simulink model "Airship_Model_2"  (R2020a)
settings: Solver=VariableStepAuto  StartTime=0.0  StopTime=300  RelTol=1e-3
values from neighbouring files (symbols this model uses):
  d = [0; 0; 0; 0; 0; 0; 0; 0; 0; 0; 0; 0]    [Inputs.m]
  g = 9.81    [Inputs.m]
  M = 997    [Inputs.m]
  rho = 0.8891    [Inputs.m]
  Sref = 6515.77    [Inputs.m]
  x0 = [0; 0; 0; 0; 0; 0; 0; 0; -20; 0; 0; 0]    [Inputs.m]
undefined symbols (not defined in the file or in its folder): sigbuilder_block
libraries: simulink x4
settings Model: Creator=roohan  LastModifiedBy=HP

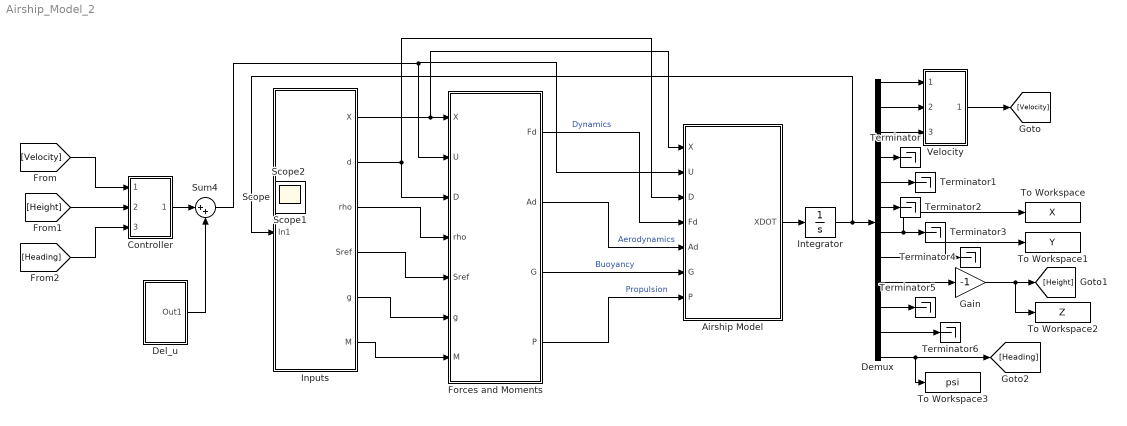
== system Airship_Model_2 ==
  Airship Model : MATLAB Function  TreatAsAtomicUnit=on
  Controller : Subsystem
  Del_u : Subsystem
  Demux : Demux  Outputs=12
  Forces and Moments : Subsystem
  Gain : Gain  Gain=-1
  Inputs : Subsystem
  Integrator : Integrator
  Sum4 : Sum  Inputs=|++
  Terminator{,1..6} (7 alike) : Terminator
  To Workspace : ToWorkspace  VariableName=X  SaveFormat=Timeseries  SampleTime=-1
  To Workspace1 : ToWorkspace  VariableName=Y  SaveFormat=Timeseries  SampleTime=-1
  To Workspace2 : ToWorkspace  VariableName=Z  SaveFormat=Timeseries  SampleTime=-1
  To Workspace3 : ToWorkspace  VariableName=psi  SaveFormat=Timeseries  SampleTime=-1
  Velocity : Subsystem
  Scope : Scope
  Scope1 : Scope
  Scope2 : Scope
  wires:
  Airship Model/1(XDOT) -> Integrator/1
  Integrator/1 -> Inputs/1(In1), Demux/1
  Forces and Moments/1(Fd) -> Airship Model/4(Fd)  "Dynamics"
  Forces and Moments/2(Ad) -> Airship Model/5(Ad)  "Aerodynamics"
  Forces and Moments/3(G) -> Airship Model/6(G)  "Buoyancy"
  Forces and Moments/4(P) -> Airship Model/7(P)  "Propulsion"
  Inputs/2(d) -> Forces and Moments/3(D), Airship Model/3(D)
  Inputs/3(rho) -> Forces and Moments/4(rho)
  Inputs/4(Sref) -> Forces and Moments/5(Sref)
  Inputs/5(g) -> Forces and Moments/6(g)
  Inputs/6(M) -> Forces and Moments/7(M)
  Inputs/1(X) -> Forces and Moments/1(X), Airship Model/1(X)
  Demux/9 -> Gain/1
  Gain/1 -> [Height], To Workspace2/1
  Demux/12 -> To Workspace3/1, [Heading]
  Sum4/1 -> Airship Model/2(U), Forces and Moments/2(U)
  Del_u/1(Out1) -> Sum4/2
  [Velocity] -> Controller/1(In1)
  [Height] -> Controller/2(In2)
  [Heading] -> Controller/3(In3)
  Controller/1(Out1) -> Sum4/1
  Demux/4 -> Terminator/1
  Demux/5 -> Terminator1/1
  Demux/6 -> Terminator2/1
  Demux/7 -> To Workspace/1, Terminator3/1
  Demux/8 -> To Workspace1/1, Terminator4/1
  Demux/10 -> Terminator5/1
  Demux/11 -> Terminator6/1
  Demux/1 -> Velocity/1(In1)
  Demux/2 -> Velocity/2(In2)
  Demux/3 -> Velocity/3(In3)
  Velocity/1(Out1) -> [Velocity]

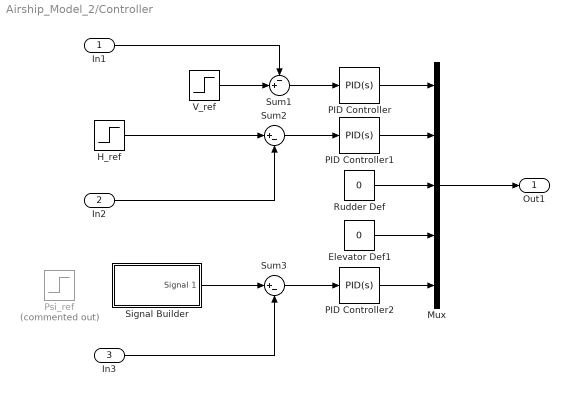
== system Airship_Model_2/Controller ==
  In1 : Inport
  In2 : Inport  Port=2
  In3 : Inport  Port=3
  Elevator Def1 : Constant  Value=0
  H_ref : Step  SampleTime=0.075
  Mux : Mux  Inputs=5
  PID Controller : simulink/Continuous/PID Controller  Controller=PID  Form=Parallel  TimeDomain=Continuous-time  UseExternalTs=off  SampleTime=-1  IntegratorMethod=Forward Euler  FilterMethod=Forward Euler  ControllerParametersSource=internal  P=15  I=0.001  D=15  UseFilter=on  N=100  TunerSelectOption=Transfer Function Based (PID Tuner App)  InitialConditionSource=internal  InitialConditionForIntegrator=0  InitialConditionForFilter=0  DifferentiatorICPrevScaledInput=0  ExternalReset=none  TrackingMode=off  Kt=1  LimitOutput=off  UpperSaturationLimit=inf  LowerSaturationLimit=-inf  LinearizeAsGain=on  AntiWindupMode=none  Kb=1  POutMin=[]  POutMax=[]  IOutMin=[]  IOutMax=[]  DOutMin=[]  DOutMax=[]  NOutMin=[]  NOutMax=[]  SumOutMin=[]  SumOutMax=[]  SaturationOutMin=[]  SaturationOutMax=[]  PParamMin=[]  PParamMax=[]  IParamMin=[]  IParamMax=[]  DParamMin=[]  DParamMax=[]  NParamMin=[]  NParamMax=[]  KbParamMin=[]  KbParamMax=[]  KtParamMin=[]  KtParamMax=[]  KbOutMin=[]  KbOutMax=[]  KtOutMin=[]  KtOutMax=[]  IntegratorOutMin=[]  IntegratorOutMax=[]  FilterOutMin=[]  FilterOutMax=[]  SumI1OutMin=[]  SumI1OutMax=[]  SumI2OutMin=[]  SumI2OutMax=[]  SumI3OutMin=[]  SumI3OutMax=[]  SumI4OutMin=[]  SumI4OutMax=[]  SumDOutMin=[]  SumDOutMax=[]  DifferentiatorOutMin=[]  DifferentiatorOutMax=[]  FilterDiffOutCoefMin=[]  FilterDiffOutCoefMax=[]  ReciprocalOutMin=[]  ReciprocalOutMax=[]  SumDenOutMin=[]  SumDenOutMax=[]  SumNumOutMin=[]  SumNumOutMax=[]  DivideOutMin=[]  DivideOutMax=[]  UdiffTsProdOutMin=[]  UdiffTsProdOutMax=[]  NTsProdOutMin=[]  NTsProdOutMax=[]  UintegralTsProdOutMin=[]  UintegralTsProdOutMax=[]  UngainTsProdOutMin=[]  UngainTsProdOutMax=[]  IntegratorContinuousStateAttributes=''  IntegratorStateMustResolveToSignalObject=off  IntegratorRTWStateStorageClass=Auto  FilterContinuousStateAttributes=''  FilterStateMustResolveToSignalObject=off  FilterRTWStateStorageClass=Auto  ParallelPVariant=InternalParameters  IdealPVariant=Disabled  IVariant=InternalParameters  DVariant=InternalParameters  IntegratorVariant=Continuous  SatVariant=Disabled  AWVariant=Passthrough  PCopyVariant=Disabled  TRVariant=Disabled  FdbkBlocksVariant=Forward  IdealPFdbkVariant=Disabled  SatFdbkVariant=Disabled  DerivativeFilterVariant=ContFilter  NVariant=InternalParameters  NCopyVariant=Disabled  FilterICVariant=InternalICsFilter  IntegratorICVariant=InternalICs  ExternalResetVariant=Disabled  TRSumVariant=Passthrough  SumFdbkVariant=Disabled  SumVariant=Sum_PID  TsampFilterVariant=InternalTs  TsampNgainVariant=Passthrough  TsampIntegralVariant=Passthrough
  PID Controller1 : simulink/Continuous/PID Controller  Controller=PID  Form=Parallel  TimeDomain=Continuous-time  UseExternalTs=off  SampleTime=-1  IntegratorMethod=Forward Euler  FilterMethod=Forward Euler  ControllerParametersSource=internal  P=3  I=0.005  D=10  UseFilter=on  N=100  TunerSelectOption=Transfer Function Based (PID Tuner App)  InitialConditionSource=internal  InitialConditionForIntegrator=0  InitialConditionForFilter=0  DifferentiatorICPrevScaledInput=0  ExternalReset=none  TrackingMode=off  Kt=1  LimitOutput=off  UpperSaturationLimit=inf  LowerSaturationLimit=-inf  LinearizeAsGain=on  AntiWindupMode=none  Kb=1  POutMin=[]  POutMax=[]  IOutMin=[]  IOutMax=[]  DOutMin=[]  DOutMax=[]  NOutMin=[]  NOutMax=[]  SumOutMin=[]  SumOutMax=[]  SaturationOutMin=[]  SaturationOutMax=[]  PParamMin=[]  PParamMax=[]  IParamMin=[]  IParamMax=[]  DParamMin=[]  DParamMax=[]  NParamMin=[]  NParamMax=[]  KbParamMin=[]  KbParamMax=[]  KtParamMin=[]  KtParamMax=[]  KbOutMin=[]  KbOutMax=[]  KtOutMin=[]  KtOutMax=[]  IntegratorOutMin=[]  IntegratorOutMax=[]  FilterOutMin=[]  FilterOutMax=[]  SumI1OutMin=[]  SumI1OutMax=[]  SumI2OutMin=[]  SumI2OutMax=[]  SumI3OutMin=[]  SumI3OutMax=[]  SumI4OutMin=[]  SumI4OutMax=[]  SumDOutMin=[]  SumDOutMax=[]  DifferentiatorOutMin=[]  DifferentiatorOutMax=[]  FilterDiffOutCoefMin=[]  FilterDiffOutCoefMax=[]  ReciprocalOutMin=[]  ReciprocalOutMax=[]  SumDenOutMin=[]  SumDenOutMax=[]  SumNumOutMin=[]  SumNumOutMax=[]  DivideOutMin=[]  DivideOutMax=[]  UdiffTsProdOutMin=[]  UdiffTsProdOutMax=[]  NTsProdOutMin=[]  NTsProdOutMax=[]  UintegralTsProdOutMin=[]  UintegralTsProdOutMax=[]  UngainTsProdOutMin=[]  UngainTsProdOutMax=[]  IntegratorContinuousStateAttributes=''  IntegratorStateMustResolveToSignalObject=off  IntegratorRTWStateStorageClass=Auto  FilterContinuousStateAttributes=''  FilterStateMustResolveToSignalObject=off  FilterRTWStateStorageClass=Auto  ParallelPVariant=InternalParameters  IdealPVariant=Disabled  IVariant=InternalParameters  DVariant=InternalParameters  IntegratorVariant=Continuous  SatVariant=Disabled  AWVariant=Passthrough  PCopyVariant=Disabled  TRVariant=Disabled  FdbkBlocksVariant=Forward  IdealPFdbkVariant=Disabled  SatFdbkVariant=Disabled  DerivativeFilterVariant=ContFilter  NVariant=InternalParameters  NCopyVariant=Disabled  FilterICVariant=InternalICsFilter  IntegratorICVariant=InternalICs  ExternalResetVariant=Disabled  TRSumVariant=Passthrough  SumFdbkVariant=Disabled  SumVariant=Sum_PID  TsampFilterVariant=InternalTs  TsampNgainVariant=Passthrough  TsampIntegralVariant=Passthrough
  PID Controller2 : simulink/Continuous/PID Controller  Controller=PID  Form=Parallel  TimeDomain=Continuous-time  UseExternalTs=off  SampleTime=-1  IntegratorMethod=Forward Euler  FilterMethod=Forward Euler  ControllerParametersSource=internal  P=-3  I=0  D=-7.5  UseFilter=on  N=100  TunerSelectOption=Transfer Function Based (PID Tuner App)  InitialConditionSource=internal  InitialConditionForIntegrator=0  InitialConditionForFilter=0  DifferentiatorICPrevScaledInput=0  ExternalReset=none  TrackingMode=off  Kt=1  LimitOutput=off  UpperSaturationLimit=inf  LowerSaturationLimit=-inf  LinearizeAsGain=on  AntiWindupMode=none  Kb=1  POutMin=[]  POutMax=[]  IOutMin=[]  IOutMax=[]  DOutMin=[]  DOutMax=[]  NOutMin=[]  NOutMax=[]  SumOutMin=[]  SumOutMax=[]  SaturationOutMin=[]  SaturationOutMax=[]  PParamMin=[]  PParamMax=[]  IParamMin=[]  IParamMax=[]  DParamMin=[]  DParamMax=[]  NParamMin=[]  NParamMax=[]  KbParamMin=[]  KbParamMax=[]  KtParamMin=[]  KtParamMax=[]  KbOutMin=[]  KbOutMax=[]  KtOutMin=[]  KtOutMax=[]  IntegratorOutMin=[]  IntegratorOutMax=[]  FilterOutMin=[]  FilterOutMax=[]  SumI1OutMin=[]  SumI1OutMax=[]  SumI2OutMin=[]  SumI2OutMax=[]  SumI3OutMin=[]  SumI3OutMax=[]  SumI4OutMin=[]  SumI4OutMax=[]  SumDOutMin=[]  SumDOutMax=[]  DifferentiatorOutMin=[]  DifferentiatorOutMax=[]  FilterDiffOutCoefMin=[]  FilterDiffOutCoefMax=[]  ReciprocalOutMin=[]  ReciprocalOutMax=[]  SumDenOutMin=[]  SumDenOutMax=[]  SumNumOutMin=[]  SumNumOutMax=[]  DivideOutMin=[]  DivideOutMax=[]  UdiffTsProdOutMin=[]  UdiffTsProdOutMax=[]  NTsProdOutMin=[]  NTsProdOutMax=[]  UintegralTsProdOutMin=[]  UintegralTsProdOutMax=[]  UngainTsProdOutMin=[]  UngainTsProdOutMax=[]  IntegratorContinuousStateAttributes=''  IntegratorStateMustResolveToSignalObject=off  IntegratorRTWStateStorageClass=Auto  FilterContinuousStateAttributes=''  FilterStateMustResolveToSignalObject=off  FilterRTWStateStorageClass=Auto  ParallelPVariant=InternalParameters  IdealPVariant=Disabled  IVariant=InternalParameters  DVariant=InternalParameters  IntegratorVariant=Continuous  SatVariant=Disabled  AWVariant=Passthrough  PCopyVariant=Disabled  TRVariant=Disabled  FdbkBlocksVariant=Forward  IdealPFdbkVariant=Disabled  SatFdbkVariant=Disabled  DerivativeFilterVariant=ContFilter  NVariant=InternalParameters  NCopyVariant=Disabled  FilterICVariant=InternalICsFilter  IntegratorICVariant=InternalICs  ExternalResetVariant=Disabled  TRSumVariant=Passthrough  SumFdbkVariant=Disabled  SumVariant=Sum_PID  TsampFilterVariant=InternalTs  TsampNgainVariant=Passthrough  TsampIntegralVariant=Passthrough
  Psi_ref : Step  Commented=on  After=1.57  SampleTime=1
  Rudder Def : Constant  Value=0
  Signal Builder : Subsystem  Tag=STV Subsys  LoadFcn=sigbuilder_block('load');  StartFcn=sigbuilder_block('start');  StopFcn=sigbuilder_block('stop');  ClipboardFcn=sigbuilder_block('clipboard');  mask(Sigbuilder block){tuvar=[0:10]}
      mask help: Simulink:masks:SigbuilderBlock_MD
      mask init:
      | if ~strcmp(get_param(bdroot(gcbh),'SimulationStatus'),'stopped') tuvar = sigbuilder_block('maskInit'); end
      settings: CopyFcn=sigbuilder_block('copy');  DeleteFcn=sigbuilder_block('delete');  ModelCloseFcn=sigbuilder_block('modelClose');  PreSaveFcn=sigbuilder_block('preSave');  PauseFcn=sigbuilder_block('pause');  ContinueFcn=sigbuilder_block('continue');  NameChangeFcn=sigbuilder_block('namechange');  OpenFcn=sigbuilder_block('open',[0 30 1024.5 488.25 ]);  CloseFcn=sigbuilder_block('close');
      mask Display: plot(0, 0, 100, 100,[2, 2, 32, 32, 2], [68, 8, 8, 68, 68],[32, 2], [38, 38], [32, 19, 2],[53, 60, 44], [32, 17, 17, 2],[16, 16, 31, 31]);txt = getActiveGroup(gcbh);text(2, 100, txt,'verticalAlignment', 'top');
  Sum1 : Sum  Inputs=-+|
  Sum2 : Sum  Inputs=|+-
  Sum3 : Sum  Inputs=|+-
  V_ref : Step  SampleTime=0.1
  Out1 : Outport
  wires:
  Sum2/1 -> PID Controller1/1
  Sum3/1 -> PID Controller2/1
  V_ref/1 -> Sum1/2
  PID Controller2/1 -> Mux/5
  PID Controller/1 -> Mux/1
  Rudder Def/1 -> Mux/3
  Sum1/1 -> PID Controller/1
  Elevator Def1/1 -> Mux/4
  PID Controller1/1 -> Mux/2
  In2/1 -> Sum2/2
  In1/1 -> Sum1/1
  In3/1 -> Sum3/2
  Mux/1 -> Out1/1
  Signal Builder/1(Signal 1) -> Sum3/1
  H_ref/1 -> Sum2/1

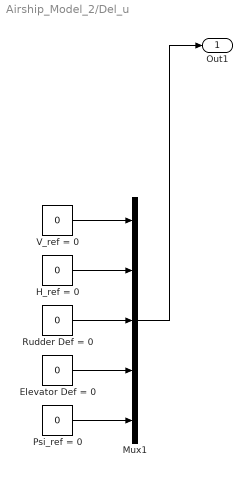
== system Airship_Model_2/Del_u ==
  Elevator Def = 0 : Constant  Value=0
  H_ref = 0 : Constant  Value=0
  Mux1 : Mux  Inputs=5
  Psi_ref = 0 : Constant  Value=0
  Rudder Def = 0 : Constant  Value=0
  V_ref = 0 : Constant  Value=0
  Out1 : Outport
  wires:
  V_ref = 0/1 -> Mux1/1
  H_ref = 0/1 -> Mux1/2
  Rudder Def = 0/1 -> Mux1/3
  Psi_ref = 0/1 -> Mux1/5
  Mux1/1 -> Out1/1
  Elevator Def = 0/1 -> Mux1/4

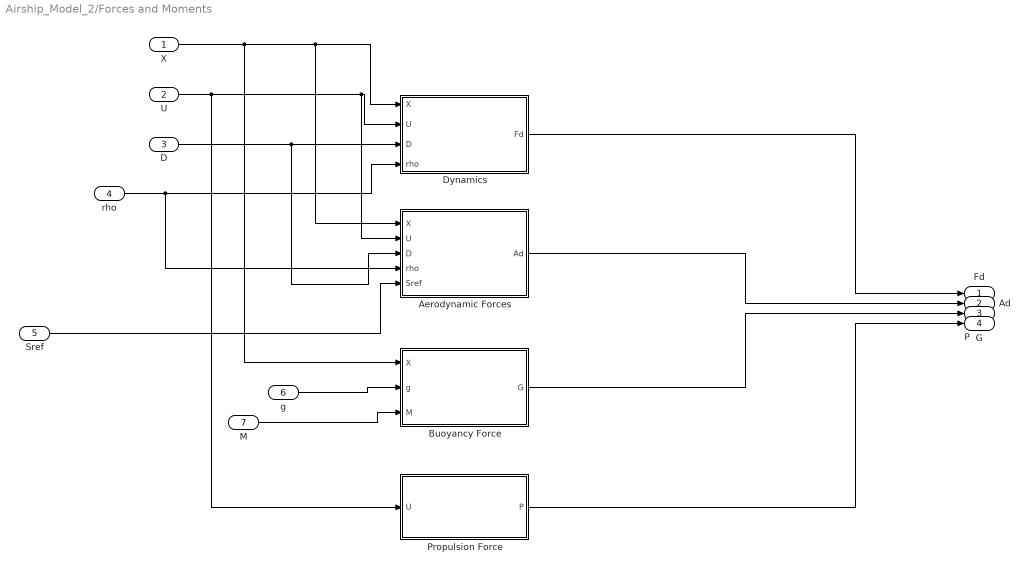
== system Airship_Model_2/Forces and Moments ==
  X : Inport
  U : Inport  Port=2
  D : Inport  Port=3
  rho : Inport  Port=4
  Sref : Inport  Port=5
  g : Inport  Port=6
  M : Inport  Port=7
  Aerodynamic Forces : MATLAB Function  TreatAsAtomicUnit=on
  Buoyancy Force : MATLAB Function  TreatAsAtomicUnit=on
  Dynamics : MATLAB Function  TreatAsAtomicUnit=on
  Propulsion Force : MATLAB Function  TreatAsAtomicUnit=on
  Fd : Outport
  Ad : Outport  Port=2
  G : Outport  Port=3
  P : Outport  Port=4
  wires:
  Buoyancy Force/1(G) -> G/1
  D/1 -> Aerodynamic Forces/3(D), Dynamics/3(D)
  X/1 -> Buoyancy Force/1(X), Dynamics/1(X), Aerodynamic Forces/1(X)
  U/1 -> Propulsion Force/1(U), Aerodynamic Forces/2(U), Dynamics/2(U)
  Aerodynamic Forces/1(Ad) -> Ad/1
  Propulsion Force/1(P) -> P/1
  g/1 -> Buoyancy Force/2(g)
  Dynamics/1(Fd) -> Fd/1
  Sref/1 -> Aerodynamic Forces/5(Sref)
  rho/1 -> Aerodynamic Forces/4(rho), Dynamics/4(rho)
  M/1 -> Buoyancy Force/3(M)

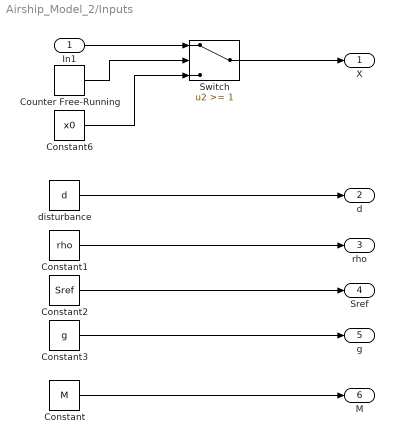
== system Airship_Model_2/Inputs ==
  In1 : Inport
  Constant : Constant  Value=M
  Constant1 : Constant  Value=rho
  Constant2 : Constant  Value=Sref
  Constant3 : Constant  Value=g
  Constant6 : Constant  Value=x0
  Counter Free-Running : simulink/Sources/Counter Free-Running  NumBits=16  tsamp=-1
  Switch : Switch  Threshold=1
  disturbance : Constant  Value=d
  X : Outport
  d : Outport  Port=2
  rho : Outport  Port=3
  Sref : Outport  Port=4
  g : Outport  Port=5
  M : Outport  Port=6
  wires:
  disturbance/1 -> d/1
  Switch/1 -> X/1
  Constant6/1 -> Switch/3
  Constant1/1 -> rho/1
  Counter Free-Running/1 -> Switch/2
  Constant2/1 -> Sref/1
  Constant3/1 -> g/1
  Constant/1 -> M/1
  In1/1 -> Switch/1

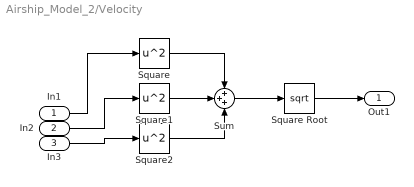
== system Airship_Model_2/Velocity ==
  In1 : Inport
  In2 : Inport  Port=2
  In3 : Inport  Port=3
  Square : Math  Operator=square  SaturateOnIntegerOverflow=on
  Square Root : Sqrt  SaturateOnIntegerOverflow=on
  Square1 : Math  Operator=square  SaturateOnIntegerOverflow=on
  Square2 : Math  Operator=square  SaturateOnIntegerOverflow=on
  Sum : Sum  Inputs=+++
  Out1 : Outport
  wires:
  In3/1 -> Square2/1
  Square1/1 -> Sum/2
  Square/1 -> Sum/1
  Square2/1 -> Sum/3
  Sum/1 -> Square Root/1
  In2/1 -> Square1/1
  In1/1 -> Square/1
  Square Root/1 -> Out1/1

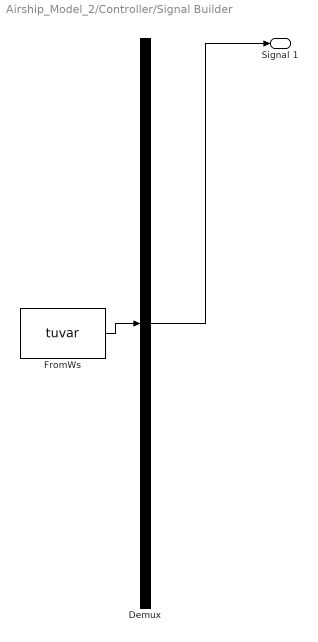
== system Airship_Model_2/Controller/Signal Builder ==
  Demux : Demux  Tag=STV Demux  Outputs=1
      settings: DisplayOption=none
  FromWs : FromWorkspace  Tag=STV FromWs  VariableName=tuvar
      SigBuilderData=|
      | common.afterFinalStr = 'Extrapolate'
      | common.sampleTime = 0
      | dataSet.timeRange = [0 300]
      | dataSet.name = 'Group 1'
      | sbobj.Groups.Name = 'Group 1'
      | sbobj.Groups.Signals.Name = 'Signal 1'
      | sbobj.Groups.Signals.XData = [0 150 150 200 200 300]
      | sbobj.Groups.Signals.YData = [0 0 0.785 0.785 0 0]
      | sbobj.Groups.TimeRange = [0 300]
  Signal 1 : Outport  Tag=STV Outport
  wires:
  Demux/1 -> Signal 1/1
  FromWs/1 -> Demux/1

== matlab function Airship_Model_2/Airship Model ==
  data: X input; XDOT output; U input; D input; Fd input; Ad input; G input; P input
function XDOT  = AIRSHIP(X,U,D, Fd, Ad, G, P)
% State Vector
x1 = X(1); % u
x2 = X(2); % v
x3 = X(3); % w
x4 = X(4); % p
x5 = X(5); % q
x6 = X(6); % r
x7 = X(7); % x
x8 = X(8); % y
x9 = X(9); % z
x10 = X(10); % phi
x11 = X(11); % theta
x12 = X(12); % psi
% Inputs
u1 = U(1); % TM
u2 = U(2); % gammaTM
u3 = U(3); % deltaE
u4 = U(4); % deltaR
u5 = U(5); % TT
% Disturbance
uw = D(1);
vw = D(2);
ww = D(3);
uw_dot = D(4);
vw_dot = D(5);
ww_dot = D(6);
pw = D(7);
qw = D(8);
rw = D(9);
pw_dot = D(10);
qw_dot = D(11);
rw_dot = D(12);
% Mass Matrix
invM = [ 0.0461 0 0.0015 0 -0.0009 0;
        0 0.0357 0 0.0163 0 0.0046;
        0.0015 0 0.0314 0 -0.0041 0;
        0 0.0163 0 0.0576 0 0.0017;
        -0.0009 0 -0.0041 0 0.0025 0;
        0 0.0046 0 0.0017 0 0.0025];
    
% Kinematics
% Rotation matrix
R11 = cos(x11)*cos(x12);
R12 = cos(x11)*sin(x12);
R13 = -sin(x11);
R21 = -cos(x10)*sin(x12) + sin(x10)*sin(x11)*cos(x12);
R22 = cos(x10)*cos(x12) + sin(x10)*sin(x11)*sin(x12);
R23 = sin(x10)*cos(x11);
R31 = sin(x10)*sin(x12) + cos(x10)*sin(x11)*cos(x12);
R32 = -sin(x10)*cos(x12) + cos(x10)*sin(x11)*sin(x12);
R33 = cos(x10)*cos(x11);
RIB = [R11 R12 R13;...
       R21 R22 R23;...
       R31 R32 R33];
% Euler angles
G11 = 1;
G12 = sin(x10)*tan(x11);
G13 = cos(x10)*tan(x11);
G21 = 0;
G22 = cos(x10);
G23 = -sin(x10);
G31 = 0;
G32 = sin(x10)/cos(x11);
G33 = cos(x10)/cos(x11);
Gamma = [G11 G12 G13;...
        G21 G22 G23;...
        G31 G32 G33];
% Wind Vector
MBa = [21.8546 0 0;
       0 41.4203 0;
       0 0 40.7490];
JBa = [19.9881 0 4.4811;
        0 520.9601 0;
       4.4811 0 526.9284];
Vw = [uw; vw; ww];
Vw_dot = [uw_dot; vw_dot; ww_dot];
omega = [x4;x5;x6];
omegaw = [pw; qw; rw];
omegaw_dot = [pw_dot; qw_dot; rw_dot];
W1to3 = MBa*Vw_dot + cross(omega, (MBa*Vw));
W4to6 = JBa*omegaw_dot + cross(omega, (JBa*omegaw));
W = [W1to3; W4to6];
% phidot, thetadot, psidot
x10to12dot = Gamma*omega;
% xdot, ydot, zdot
Vvec = [x1;x2;x3];
x7to9dot = (RIB.')*Vvec;
% Dynamics
x1to6dot = invM*(Fd + Ad + G + P + W);
% XDOT
XDOT = [x1to6dot; x7to9dot; x10to12dot];

== matlab function Airship_Model_2/Forces and Moments/Propulsion Force ==
  data: U input; P output
function P = Propulsion(U)
    % Extract inputs
    u1 = U(1);
    u2 = U(2);
    u5 = U(5);

    % Define propulsion calculations
    mx = -0.31; my = 0; mz = 1.1; % Main thruster
    tx = -3.29; ty = 0; tz = -0.25; % Tail thruster 
   
    Xp = u1*cos(u2);
    Yp = u5;
    Zp = -u1*sin(u2);
    Lp = -(u5*tz);
    Mp = u1*mz*cos(u2) - u1*mx*sin(u2);
    Np = (u5*tx);

    P = [Xp; Yp; Zp; Lp; Mp; Np];
end

== matlab function Airship_Model_2/Forces and Moments/Aerodynamic Forces ==
  data: X input; Ad output; U input; D input; rho input; Sref input
function Ad = Aerodynamics(X, U, D, rho, Sref)
    
    % Disturbance
    uw = D(1);
    vw = D(2);
    ww = D(3);
    % Inputs
    u1 = U(1); % TM
    u2 = U(2); % gammaTM
    u3 = U(3); % deltaE
    u4 = U(4); % deltaR
    u5 = U(5); % TT
    % Extract variables dependent upon states
    Vmag = sqrt(X(1)^2 + X(2)^2 + X(3)^2);
    Vw_mag = sqrt(uw^2 + vw^2 + ww^2);
    Va = Vmag - Vw_mag;
    alpha = atan2(X(3),X(1));
    beta = atan2(X(2)*cos(alpha), X(1));
    
    % Define aerodynamic calculations
    CX1 = -0.0789; CX2 = -0.7769;
    CY1 = CX2; CY2 = -0.4154; CY3 = -1.7211; CY4 = 0.0899;
    CZ1 = CX2; CZ2 = CY2; CZ3 = -1.2211; CZ4 = -CY4;
    CL2 = 0;
    CM1 = 2.2194; CM2 = -1.4789; CM3 = -0.4816; CM4 = -0.1291;
    CN1 = -CM1; CN2 = -CM2; CN3 = -CM3; CN4 = CM4;
    AX = 0.5*rho*Va^2*(CX1*cos(alpha)^2*cos(beta)^2 + CX2*sin(2*alpha)*sin(alpha/2));
    AY = 0.5*rho*Va^2*(CY1*cos(beta/2)*sin(2*beta) + CY2*sin(2*beta) + CY3*sin(beta)*sin(abs(beta)) + 2*CY4*u4);
    AZ = 0.5*rho*Va^2*(CZ1*cos(alpha/2)*sin(2*alpha) + CZ2*sin(2*alpha) +CZ3*sin(alpha)*sin(abs(alpha)) + 2*CZ4*u3);
    AL = 0.5*rho*Va^2*(CL2*sin(beta)*sin(abs(beta)));
    AM = 0.5*rho*Va^2*(CM1*cos(alpha/2)*sin(2*alpha) + CM2*sin(2*alpha) + CM3*sin(alpha)*sin(abs(alpha)) + 2*CM4*u3);
    AN = 0.5*rho*Va^2*(CN1*cos(beta/2)*sin(2*beta) + CN2*sin(2*beta) + CN3*sin(beta)*sin(abs(beta)) + 2*CN4*u4);
    Ad = [AX; AY; AZ; AL; AM; AN];
end

== matlab function Airship_Model_2/Forces and Moments/Buoyancy Force ==
  data: X input; G output; g input; M input
function G = Buoyancy(X, g, M)
    % Extract inputs
  
    x1 = X(1); % u
    x2 = X(2); % v
    x3 = X(3); % w
    x4 = X(4); % p
    x5 = X(5); % q
    x6 = X(6); % r
    x7 = X(7); % x
    x8 = X(8); % y
    x9 = X(9); % z
    x10 = X(10); % phi
    x11 = X(11); % theta
    x12 = X(12); % psi
    
    ax = 0; ay = 0; az = 0.4032; % CM
    bx = 0; by = 0; bz = 0; % CV
    
    Fg = M*g;
    Fb = Fg; % neutral buoyancy
    Xgb = -(Fg - Fb)*sin(x11);
    Ygb = (Fg - Fb)*sin(x10)*cos(x11);
    Zgb = (Fg - Fb)*cos(x10)*cos(x11);
    Lgb = -(Fg*az - Fb*bz)*cos(x11)*sin(x10);
    Mgb = -((Fg*az + Fb*bz)*sin(x11)) - ((Fg*ax + Fb*bx)*cos(x11)*cos(x10));
    Ngb = (Fg*ax + Fb*bx)*sin(x10)*cos(x11);

    G = [Xgb; Ygb; Zgb; Lgb; Mgb; Ngb];
end

== matlab function Airship_Model_2/Forces and Moments/Dynamics ==
  data: X input; Fd output; U input; D input; rho input
function Fd = Dynamics(X, U, D, rho)
% State Vector
x1 = X(1); % u
x2 = X(2); % v
x3 = X(3); % w
x4 = X(4); % p
x5 = X(5); % q
x6 = X(6); % r
x7 = X(7); % x
x8 = X(8); % y
x9 = X(9); % z
x10 = X(10); % phi
x11 = X(11); % theta
x12 = X(12); % psi
% Inputs
u1 = U(1); % TM
u2 = U(2); % gammaTM
u3 = U(3); % deltaE
u4 = U(4); % deltaR
u5 = U(5); % TT
% Disturbance
uw = D(1);
vw = D(2);
ww = D(3);
uw_dot = D(4);
vw_dot = D(5);
ww_dot = D(6);
pw = D(7);
qw = D(8);
rw = D(9);
pw_dot = D(10);
qw_dot = D(11);
rw_dot = D(12);
% Dynamics Vector
a11 = 1.247*rho;
a22 = 17.219*rho;
a26 = -56.893*rho;
a35 = 55.269*rho;
a15 = 0;
a24 = -1.231*rho;
a33 = 16.671*rho;
a42 = a24;
a44 = 13.38*rho;
a51 = a15;
a55 = 311.942*rho;
a46 = 3.658*rho;
a64 = a46;
a53 = a35;
a62 = a26;
a66 = 316.814*rho;
m13 = 1.045*rho;
m33 = -40.573*rho;
xm11 = 20.973*rho;
xm22 = 19.337*rho;
xm13 = -3.721*rho;
x2m11 = -141.625*rho;
x2m22 = -135.799*rho;
D11 = 0;
D12 = a22*x6;
D13 = -a33*x5;
D14 = a24*x6;
D15 = -a35*x5;
D16 = a26*x6;
D21 = x4*m13 + x6*(xm11-a11);
D22 = 0;
D23 =a33*x4;
D24 = a35*x5;
D25 = -a15*x5;
D26 = 0;
D31 = (a11-xm22)*x5;
D32 = -a22*x4;
D33 = 0;
D34 = -(a24*x4) - (a26*x6);
D35 = a15*x5;
D36 = 0;
D41 = x4*m33 + x6*(a15+xm13);
D42 = -(a62+a35)*x5;
D43 = (a62+a35)*x6 + a24*x4;
D44 = -a64*x5;
D45 =(a55-a66)*x6;
D46 = 0;
D51 = (a35+x2m22)*x5;
D52 = -a42*x6 + a62*x4;
D53 = -a15*x5;
D54 = a64*x4 + (a66-a44)*x6;
D55 = 0;
D56 = -a64*x6;
D61 = -(a51+a24-xm13)*x4 - (a26-x2m11)*x6;
D62 = (a15+a42)*x5;
D63 = -a53*x4;
D64 = (a44- a55)*x5;
D65 = a46*x6;
D66 = 0;
D = [D11 D12 D13 D14 D15 D16;...
    D21 D22 D23 D24 D25 D26;...
    D31 D32 D33 D34 D35 D36;...
    D41 D42 D43 D44 D45 D46;...
    D51 D52 D53 D54 D55 D56;...
    D61 D62 D63 D64 D65 D66];
Fd = D*[x1; x2; x3; x4; x5; x6];
end
